simulink library "Float"  (R2019a)
settings: Solver=VariableStepAuto  StartTime=0.0  StopTime=10.0  RelTol=1e-3
libraries: arduinolib x2, $bdroot x2, dspstat3 x2
settings Model: Creator=Peter  LastModifiedBy=Gergely

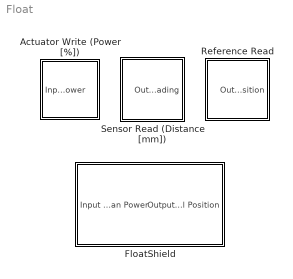
== system Float ==
  Actuator Write (Power [%]) : Subsystem
      mask DialogControl DescGroupVar Prompt: FloatShield Fan
      mask DialogControl DescTextVar Prompt: Sets power level to the rotating fan at the bottom of the FloatShield tube. Expects input in the range of 0-100%
      mask Display: image('assets\Fan.svg');
  FloatShield : Subsystem  mask{Tcal=5, Ts=0.025}
      mask prompts: Tcal "Calibration time (s):"; Ts "Sampling period (s):"
      mask DialogControl DescGroupVar Prompt: FloatShield
      mask DialogControl DescTextVar Prompt: The block represents the FloatShield device. It accepts an input signal in the range of 0-100% that controls the fan power level and outputs distance sensor reading in the range scaled to 0-100%. The block requires a sampling period and a calibration time at the beginning of the experiment to find out the reading extreme values.
      mask Display: image('assets\FloatShield.svg');
  Reference Read : Subsystem  mask{ReadoutRadio=Percentage, Ts=0.025}
      mask prompts: ReadoutRadio "Readout type"; Ts "Sample time (s):"
      mask init:
      | if ReadoutRadio==1 
      | ADC_Gain=(100.0/1023);    % Percentage
      |                                 
      | elseif ReadoutRadio==2
      | ADC_Gain=(5.0/1023);      % Voltage
      |                       
      | else
      | ADC_Gain=1.0;             % ADC levels
      | end
      mask TypeOptions ReadoutRadio: Percentage | Voltage | ADC levels
      mask DialogControl DescGroupVar Prompt: FloatShield Potentiometer
      mask DialogControl DescTextVar Prompt: The block represents the potentiometer on the FloatShield device. Based on the users choice, block outputs different forms of potentiometer actual position.
      mask Display: image('assets\Potentiometer.svg');
  Sensor Read (Distance [mm]) : Subsystem  mask{Ts=0.025}
      mask prompts: Ts "Sample Time (s):"
      mask DialogControl DescGroupVar Prompt: FloatShield Distance Sensor
      mask DialogControl DescTextVar Prompt: The block represents the I2C Time of Flight VL53L0X Distance Sensor on the FloatShield device. Periodically outputs raw distance reading from sensor in millimetres with specified sample time.
      mask Display: image('assets\TOF.svg');

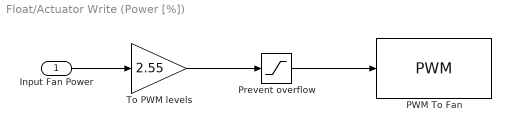
== system Float/Actuator Write (Power [%]) ==
  Input Fan Power : Inport
  PWM To Fan : arduinolib/PWM  pinNumber=3  EnableInputFrequency=off  InitialFrequency=2000  InitialDutyCycle=0  NotificationType=None  blockPlatform=arduino
  Prevent overflow : Saturate  UpperLimit=255  LowerLimit=0
  To PWM levels : Gain  Gain=2.55
  wires:
  Prevent overflow/1 -> PWM To Fan/1
  To PWM levels/1 -> Prevent overflow/1
  Input Fan Power/1 -> To PWM levels/1

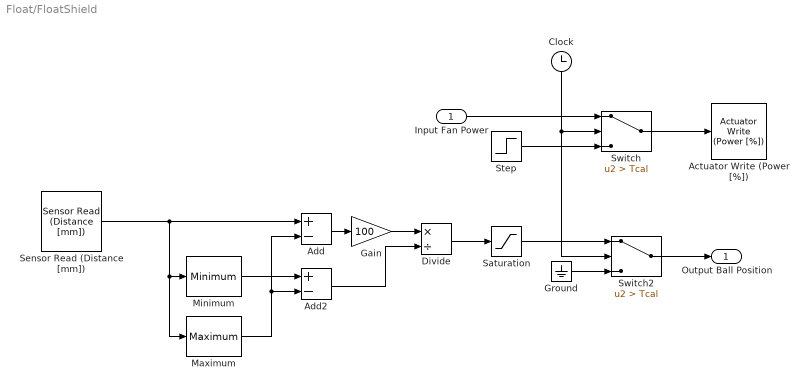
== system Float/FloatShield ==
  Input Fan Power : Inport
  Actuator Write (Power [%]) : $bdroot/Actuator Write (Power [%])
  Add : Sum  Inputs=+-
  Add2 : Sum  Inputs=+-
  Clock : Clock
  Divide : Product  Inputs=*/
  Gain : Gain  Gain=100
  Ground : Ground
  Maximum : dspstat3/Maximum  operation=maximum  fcn=Running  indexBase=One  operateOver=Each column  Dimension=1  reset=None  roiEnable=off  roiType=Rectangles  roiPortion=Entire ROI  roiOutput=Individual statistics for each ROI  roiFlag=off  roundingMode=Floor  overflowMode=off  accumDataTypeStr=Inherit: Same as product output  accumLastDataTypeStr=Inherit: Same as product output
  Minimum : dspstat3/Minimum  operation=minimum  fcn=Running  indexBase=One  operateOver=Each column  Dimension=1  reset=None  roiEnable=off  roiType=Rectangles  roiPortion=Entire ROI  roiOutput=Individual statistics for each ROI  roiFlag=off  roundingMode=Floor  overflowMode=off
      settings: SourceProductName=DSP System Toolbox  SourceProductBaseCode=DS
  Saturation : Saturate  UpperLimit=100  LowerLimit=0
  Sensor Read (Distance [mm]) : $bdroot/Sensor Read (Distance [mm])  Ts=0.025
  Step : Step  Time=round((Tcal/2)/Ts)*Ts  After=100  SampleTime=Ts
  Switch : Switch  Criteria=u2 > Threshold  Threshold=Tcal
  Switch2 : Switch  Criteria=u2 > Threshold  Threshold=Tcal
  Output Ball Position : Outport
  wires:
  Maximum/1 -> Add/2, Add2/2
  Gain/1 -> Divide/1
  Clock/1 -> Switch2/2, Switch/2
  Sensor Read (Distance [mm])/1 -> Add/1, Maximum/1, Minimum/1
  Step/1 -> Switch/3
  Minimum/1 -> Add2/1
  Add2/1 -> Divide/2
  Switch/1 -> Actuator Write (Power [%])/1
  Switch2/1 -> Output Ball Position/1
  Input Fan Power/1 -> Switch/1
  Divide/1 -> Saturation/1
  Saturation/1 -> Switch2/1
  Add/1 -> Gain/1
  Ground/1 -> Switch2/3

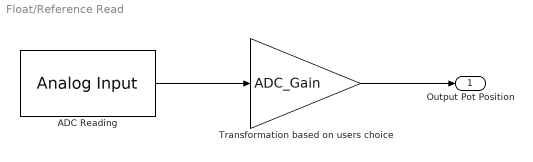
== system Float/Reference Read ==
  ADC Reading : arduinolib/Analog Input  pinNumber=0  ReadResultsOnly=off  ConversionTriggerSource=Software  ExternalTriggerType=uint32(0)  OutputDataType=uint16  EnableConversionCompleteNotify=off  EnableOuputStatus=off  SampleTime=Ts  blockPlatform=arduino
  Transformation based on users choice : Gain  Gain=ADC_Gain
  "Output Pot Position " : Outport
  wires:
  ADC Reading/1 -> Transformation based on users choice/1
  Transformation based on users choice/1 -> "Output Pot Position "/1

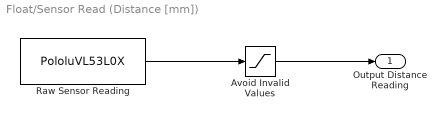
== system Float/Sensor Read (Distance [mm]) ==
  Avoid Invalid Values : Saturate  UpperLimit=345  LowerLimit=15
  Raw Sensor Reading : S-Function  FunctionName=PololuVL53L0X  SFunctionModules='PololuVL53L0X_wrapper'  SFunctionDeploymentMode=off  EnableBusSupport=off
  Output Distance Reading : Outport  SampleTime=Ts
  wires:
  Raw Sensor Reading/1 -> Avoid Invalid Values/1
  Avoid Invalid Values/1 -> Output Distance Reading/1
